simulink model "AN_Simulink_Model_v1_fil"  (R2019b)
settings: Solver=VariableStepAuto  StartTime=0.0  StopTime=testtime  RelTol=1e-3
InitFcn:
  | AN_InitFcn_Callback
StopFcn:
  | AN_StopFcn_Callback
values from neighbouring files (symbols this model uses):
  tdres = 1/Fs    (= 2.08333333333e-05)    [AN_Set_Model_Parameters.m]
libraries: hdlmdlgenlib x163, simulink x4, fillib x1, dspsrcs4 x1
(part 3 of 5)

== system AN_Simulink_Model_v1_fil/Auditory Nerve Model/C2 Wideband Filter/Sum7 ==
  In1 : Inport
  In2 : Inport  Port=2
  Sum7 : Sum  OutDataTypeStr=single  SampleTime=2.08333333333333e-05  SaturateOnIntegerOverflow=on  InputSameDT=on
  Out1 : Outport
  wires:
  Sum7/1 -> Out1/1
  In2/1 -> Sum7/2
  In1/1 -> Sum7/1

== system AN_Simulink_Model_v1_fil/Auditory Nerve Model/C2 Wideband Filter/Sum8 ==
  In1 : Inport
  In2 : Inport  Port=2
  Sum8 : Sum  OutDataTypeStr=single  SampleTime=2.08333333333333e-05  SaturateOnIntegerOverflow=on  InputSameDT=on
  Out1 : Outport
  wires:
  Sum8/1 -> Out1/1
  In2/1 -> Sum8/2
  In1/1 -> Sum8/1

== system AN_Simulink_Model_v1_fil/Auditory Nerve Model/C2 Wideband Filter/Sum9 ==
  In1 : Inport
  In2 : Inport  Port=2
  Sum9 : Sum  OutDataTypeStr=single  SampleTime=2.08333333333333e-05  SaturateOnIntegerOverflow=on  InputSameDT=on
  Out1 : Outport
  wires:
  Sum9/1 -> Out1/1
  In2/1 -> Sum9/2
  In1/1 -> Sum9/1

== system AN_Simulink_Model_v1_fil/Auditory Nerve Model/Middle Ear Filter/Gain1_unaryminus ==
  In1 : Inport
  Gain1_unaryminus : UnaryMinus  SampleTime=2.08333333333333e-05
  Out1 : Outport
  wires:
  Gain1_unaryminus/1 -> Out1/1
  In1/1 -> Gain1_unaryminus/1

== system AN_Simulink_Model_v1_fil/Auditory Nerve Model/Middle Ear Filter/Gain2_unaryminus ==
  In1 : Inport
  Gain2_unaryminus : UnaryMinus  SampleTime=2.08333333333333e-05
  Out1 : Outport
  wires:
  Gain2_unaryminus/1 -> Out1/1
  In1/1 -> Gain2_unaryminus/1

== system AN_Simulink_Model_v1_fil/Auditory Nerve Model/Middle Ear Filter/Gain3_unaryminus ==
  In1 : Inport
  Gain3_unaryminus : UnaryMinus  SampleTime=2.08333333333333e-05
  Out1 : Outport
  wires:
  Gain3_unaryminus/1 -> Out1/1
  In1/1 -> Gain3_unaryminus/1

== system AN_Simulink_Model_v1_fil/Auditory Nerve Model/Middle Ear Filter/Gain5_unaryminus ==
  In1 : Inport
  Gain5_unaryminus : UnaryMinus  SampleTime=2.08333333333333e-05
  Out1 : Outport
  wires:
  Gain5_unaryminus/1 -> Out1/1
  In1/1 -> Gain5_unaryminus/1

== system AN_Simulink_Model_v1_fil/Auditory Nerve Model/Middle Ear Filter/Gain7_unaryminus ==
  In1 : Inport
  Gain7_unaryminus : UnaryMinus  SampleTime=2.08333333333333e-05
  Out1 : Outport
  wires:
  Gain7_unaryminus/1 -> Out1/1
  In1/1 -> Gain7_unaryminus/1

== system AN_Simulink_Model_v1_fil/Auditory Nerve Model/Middle Ear Filter/Gain8_unaryminus ==
  In1 : Inport
  Gain8_unaryminus : UnaryMinus  SampleTime=2.08333333333333e-05
  Out1 : Outport
  wires:
  Gain8_unaryminus/1 -> Out1/1
  In1/1 -> Gain8_unaryminus/1

== system AN_Simulink_Model_v1_fil/Auditory Nerve Model/Middle Ear Filter/Product ==
  In1 : Inport
  In2 : Inport  Port=2
  Product : Product  Inputs=**  OutDataTypeStr=single  SampleTime=2.08333333333333e-05
  Out1 : Outport
  wires:
  Product/1 -> Out1/1
  In2/1 -> Product/2
  In1/1 -> Product/1

== system AN_Simulink_Model_v1_fil/Auditory Nerve Model/Middle Ear Filter/Product1 ==
  In1 : Inport
  In2 : Inport  Port=2
  Product1 : Product  Inputs=**  OutDataTypeStr=single  SampleTime=2.08333333333333e-05
  Out1 : Outport
  wires:
  Product1/1 -> Out1/1
  In2/1 -> Product1/2
  In1/1 -> Product1/1

== system AN_Simulink_Model_v1_fil/Auditory Nerve Model/Middle Ear Filter/Product10 ==
  In1 : Inport
  In2 : Inport  Port=2
  Product10 : Product  Inputs=**  OutDataTypeStr=single  SampleTime=2.08333333333333e-05
  Out1 : Outport
  wires:
  Product10/1 -> Out1/1
  In2/1 -> Product10/2
  In1/1 -> Product10/1

== system AN_Simulink_Model_v1_fil/Auditory Nerve Model/Middle Ear Filter/Product11 ==
  In1 : Inport
  In2 : Inport  Port=2
  Product11 : Product  Inputs=**  OutDataTypeStr=single  SampleTime=2.08333333333333e-05
  Out1 : Outport
  wires:
  Product11/1 -> Out1/1
  In2/1 -> Product11/2
  In1/1 -> Product11/1

== system AN_Simulink_Model_v1_fil/Auditory Nerve Model/Middle Ear Filter/Product12 ==
  In1 : Inport
  In2 : Inport  Port=2
  Product12 : Product  Inputs=**  OutDataTypeStr=single  SampleTime=2.08333333333333e-05
  Out1 : Outport
  wires:
  Product12/1 -> Out1/1
  In2/1 -> Product12/2
  In1/1 -> Product12/1

== system AN_Simulink_Model_v1_fil/Auditory Nerve Model/Middle Ear Filter/Product13 ==
  In1 : Inport
  In2 : Inport  Port=2
  Product13 : Product  Inputs=**  OutDataTypeStr=single  SampleTime=2.08333333333333e-05
  Out1 : Outport
  wires:
  Product13/1 -> Out1/1
  In2/1 -> Product13/2
  In1/1 -> Product13/1

== system AN_Simulink_Model_v1_fil/Auditory Nerve Model/Middle Ear Filter/Product14 ==
  In1 : Inport
  In2 : Inport  Port=2
  Product14 : Product  Inputs=**  OutDataTypeStr=single  SampleTime=2.08333333333333e-05
  Out1 : Outport
  wires:
  Product14/1 -> Out1/1
  In2/1 -> Product14/2
  In1/1 -> Product14/1

== system AN_Simulink_Model_v1_fil/Auditory Nerve Model/Middle Ear Filter/Product15_to_gain ==
  In1 : Inport
  Product15_to_gain : Gain  Gain=single(0.5)
  Out1 : Outport
  wires:
  Product15_to_gain/1 -> Out1/1
  In1/1 -> Product15_to_gain/1

== system AN_Simulink_Model_v1_fil/Auditory Nerve Model/Middle Ear Filter/Product2 ==
  In1 : Inport
  In2 : Inport  Port=2
  Product2 : Product  Inputs=**  OutDataTypeStr=single  SampleTime=2.08333333333333e-05
  Out1 : Outport
  wires:
  Product2/1 -> Out1/1
  In2/1 -> Product2/2
  In1/1 -> Product2/1

== system AN_Simulink_Model_v1_fil/Auditory Nerve Model/Middle Ear Filter/Product3 ==
  In1 : Inport
  In2 : Inport  Port=2
  Product3 : Product  Inputs=**  OutDataTypeStr=single  SampleTime=2.08333333333333e-05
  Out1 : Outport
  wires:
  Product3/1 -> Out1/1
  In2/1 -> Product3/2
  In1/1 -> Product3/1

== system AN_Simulink_Model_v1_fil/Auditory Nerve Model/Middle Ear Filter/Product4 ==
  In1 : Inport
  In2 : Inport  Port=2
  Product4 : Product  Inputs=**  OutDataTypeStr=single  SampleTime=2.08333333333333e-05
  Out1 : Outport
  wires:
  Product4/1 -> Out1/1
  In2/1 -> Product4/2
  In1/1 -> Product4/1

== system AN_Simulink_Model_v1_fil/Auditory Nerve Model/Middle Ear Filter/Product5 ==
  In1 : Inport
  In2 : Inport  Port=2
  Product5 : Product  Inputs=**  OutDataTypeStr=single  SampleTime=2.08333333333333e-05
  Out1 : Outport
  wires:
  Product5/1 -> Out1/1
  In2/1 -> Product5/2
  In1/1 -> Product5/1

== system AN_Simulink_Model_v1_fil/Auditory Nerve Model/Middle Ear Filter/Product6 ==
  In1 : Inport
  In2 : Inport  Port=2
  Product6 : Product  Inputs=**  OutDataTypeStr=single  SampleTime=2.08333333333333e-05
  Out1 : Outport
  wires:
  Product6/1 -> Out1/1
  In2/1 -> Product6/2
  In1/1 -> Product6/1

== system AN_Simulink_Model_v1_fil/Auditory Nerve Model/Middle Ear Filter/Product7 ==
  In1 : Inport
  In2 : Inport  Port=2
  Product7 : Product  Inputs=**  OutDataTypeStr=single  SampleTime=2.08333333333333e-05
  Out1 : Outport
  wires:
  Product7/1 -> Out1/1
  In2/1 -> Product7/2
  In1/1 -> Product7/1

== system AN_Simulink_Model_v1_fil/Auditory Nerve Model/Middle Ear Filter/Product8 ==
  In1 : Inport
  In2 : Inport  Port=2
  Product8 : Product  Inputs=**  OutDataTypeStr=single  SampleTime=2.08333333333333e-05
  Out1 : Outport
  wires:
  Product8/1 -> Out1/1
  In2/1 -> Product8/2
  In1/1 -> Product8/1

== system AN_Simulink_Model_v1_fil/Auditory Nerve Model/Middle Ear Filter/Product9 ==
  In1 : Inport
  In2 : Inport  Port=2
  Product9 : Product  Inputs=**  OutDataTypeStr=single  SampleTime=2.08333333333333e-05
  Out1 : Outport
  wires:
  Product9/1 -> Out1/1
  In2/1 -> Product9/2
  In1/1 -> Product9/1

== system AN_Simulink_Model_v1_fil/Auditory Nerve Model/Middle Ear Filter/Sum ==
  In1 : Inport
  In2 : Inport  Port=2
  Sum : Sum  OutDataTypeStr=single  SampleTime=2.08333333333333e-05  SaturateOnIntegerOverflow=on  InputSameDT=on
  Out1 : Outport
  wires:
  Sum/1 -> Out1/1
  In2/1 -> Sum/2
  In1/1 -> Sum/1

== system AN_Simulink_Model_v1_fil/Auditory Nerve Model/Middle Ear Filter/Sum1 ==
  In1 : Inport
  In2 : Inport  Port=2
  Sum1 : Sum  OutDataTypeStr=single  SampleTime=2.08333333333333e-05  SaturateOnIntegerOverflow=on  InputSameDT=on
  Out1 : Outport
  wires:
  Sum1/1 -> Out1/1
  In2/1 -> Sum1/2
  In1/1 -> Sum1/1

== system AN_Simulink_Model_v1_fil/Auditory Nerve Model/Middle Ear Filter/Sum10 ==
  In1 : Inport
  In2 : Inport  Port=2
  Sum10 : Sum  OutDataTypeStr=single  SampleTime=2.08333333333333e-05  SaturateOnIntegerOverflow=on  InputSameDT=on
  Out1 : Outport
  wires:
  Sum10/1 -> Out1/1
  In2/1 -> Sum10/2
  In1/1 -> Sum10/1

== system AN_Simulink_Model_v1_fil/Auditory Nerve Model/Middle Ear Filter/Sum11 ==
  In1 : Inport
  In2 : Inport  Port=2
  Sum11 : Sum  OutDataTypeStr=single  SampleTime=2.08333333333333e-05  SaturateOnIntegerOverflow=on  InputSameDT=on
  Out1 : Outport
  wires:
  Sum11/1 -> Out1/1
  In2/1 -> Sum11/2
  In1/1 -> Sum11/1

== system AN_Simulink_Model_v1_fil/Auditory Nerve Model/Middle Ear Filter/Sum2 ==
  In1 : Inport
  In2 : Inport  Port=2
  Sum2 : Sum  OutDataTypeStr=single  SampleTime=2.08333333333333e-05  SaturateOnIntegerOverflow=on  InputSameDT=on
  Out1 : Outport
  wires:
  Sum2/1 -> Out1/1
  In2/1 -> Sum2/2
  In1/1 -> Sum2/1

== system AN_Simulink_Model_v1_fil/Auditory Nerve Model/Middle Ear Filter/Sum3 ==
  In1 : Inport
  In2 : Inport  Port=2
  Sum3 : Sum  OutDataTypeStr=single  SampleTime=2.08333333333333e-05  SaturateOnIntegerOverflow=on  InputSameDT=on
  Out1 : Outport
  wires:
  Sum3/1 -> Out1/1
  In2/1 -> Sum3/2
  In1/1 -> Sum3/1

== system AN_Simulink_Model_v1_fil/Auditory Nerve Model/Middle Ear Filter/Sum4 ==
  In1 : Inport
  In2 : Inport  Port=2
  Sum4 : Sum  OutDataTypeStr=single  SampleTime=2.08333333333333e-05  SaturateOnIntegerOverflow=on  InputSameDT=on
  Out1 : Outport
  wires:
  Sum4/1 -> Out1/1
  In2/1 -> Sum4/2
  In1/1 -> Sum4/1

== system AN_Simulink_Model_v1_fil/Auditory Nerve Model/Middle Ear Filter/Sum5 ==
  In1 : Inport
  In2 : Inport  Port=2
  Sum5 : Sum  OutDataTypeStr=single  SampleTime=2.08333333333333e-05  SaturateOnIntegerOverflow=on  InputSameDT=on
  Out1 : Outport
  wires:
  Sum5/1 -> Out1/1
  In2/1 -> Sum5/2
  In1/1 -> Sum5/1

== system AN_Simulink_Model_v1_fil/Auditory Nerve Model/Middle Ear Filter/Sum6 ==
  In1 : Inport
  In2 : Inport  Port=2
  Sum6 : Sum  OutDataTypeStr=single  SampleTime=2.08333333333333e-05  SaturateOnIntegerOverflow=on  InputSameDT=on
  Out1 : Outport
  wires:
  Sum6/1 -> Out1/1
  In2/1 -> Sum6/2
  In1/1 -> Sum6/1

== system AN_Simulink_Model_v1_fil/Auditory Nerve Model/Middle Ear Filter/Sum7 ==
  In1 : Inport
  In2 : Inport  Port=2
  Sum7 : Sum  OutDataTypeStr=single  SampleTime=2.08333333333333e-05  SaturateOnIntegerOverflow=on  InputSameDT=on
  Out1 : Outport
  wires:
  Sum7/1 -> Out1/1
  In2/1 -> Sum7/2
  In1/1 -> Sum7/1

== system AN_Simulink_Model_v1_fil/Auditory Nerve Model/Middle Ear Filter/Sum8 ==
  In1 : Inport
  In2 : Inport  Port=2
  Sum8 : Sum  OutDataTypeStr=single  SampleTime=2.08333333333333e-05  SaturateOnIntegerOverflow=on  InputSameDT=on
  Out1 : Outport
  wires:
  Sum8/1 -> Out1/1
  In2/1 -> Sum8/2
  In1/1 -> Sum8/1

== system AN_Simulink_Model_v1_fil/Auditory Nerve Model/Middle Ear Filter/Sum9 ==
  In1 : Inport
  In2 : Inport  Port=2
  Sum9 : Sum  OutDataTypeStr=single  SampleTime=2.08333333333333e-05  SaturateOnIntegerOverflow=on  InputSameDT=on
  Out1 : Outport
  wires:
  Sum9/1 -> Out1/1
  In2/1 -> Sum9/2
  In1/1 -> Sum9/1

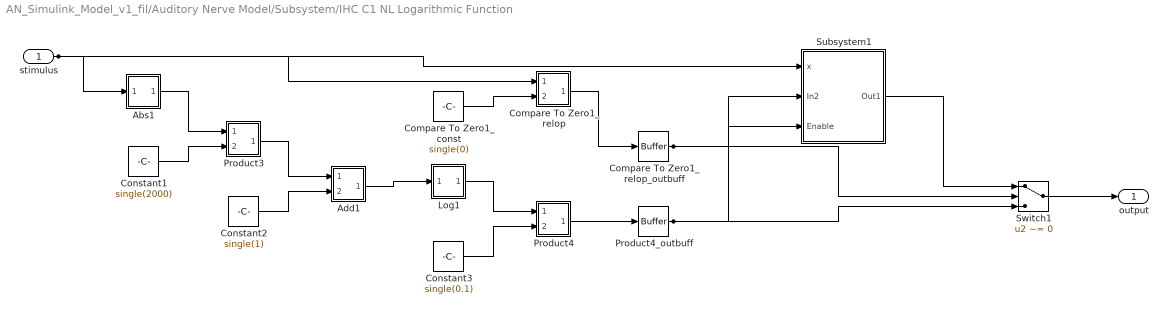
== system AN_Simulink_Model_v1_fil/Auditory Nerve Model/Subsystem/IHC C1 NL Logarithmic Function ==
  stimulus : Inport  OutDataTypeStr=single  PortDimensions=1  SampleTime=2.08333333333333e-05
  Abs1 : Subsystem
      mask Display: disp('NFP\nabs');
  Add1 : Subsystem
      mask Display: disp('NFP\nadd');
  Compare To Zero1_const : Constant  Value=single(0)  OutDataTypeStr=single  SampleTime=-1
  Compare To Zero1_relop : Subsystem
      mask Display: disp('NFP\nrelop');
  Compare To Zero1_relop_outbuff : hdlmdlgenlib/Buffer
      settings: SourceProductName=Simulink  SourceProductBaseCode=SL
  Constant1 : Constant  Value=single(2000)  OutDataTypeStr=single  SampleTime=-1
  Constant2 : Constant  Value=single(1)  OutDataTypeStr=single  SampleTime=-1
  Constant3 : Constant  Value=single(0.1)  OutDataTypeStr=single  SampleTime=-1
  Log1 : Subsystem
      mask Display: disp('NFP\nmath');
  Product3 : Subsystem
      mask Display: disp('NFP\nmul');
  Product4 : Subsystem
      mask Display: disp('NFP\nmul');
  Product4_outbuff : hdlmdlgenlib/Buffer
      settings: SourceProductName=Simulink  SourceProductBaseCode=SL
  Subsystem1 : Subsystem
  Switch1 : Switch  Criteria=u2 ~= 0  Threshold=double(0)  OutDataTypeStr=single  SampleTime=2.08333333333333e-05
  output : Outport  VectorParamsAs1DForOutWhenUnconnected=off
  wires:
  Product4/1(Out1) -> Product4_outbuff/1
  Product3/1(Out1) -> Add1/1(In1)
  Log1/1(Out1) -> Product4/1(In1)
  Compare To Zero1_relop/1(Out1) -> Compare To Zero1_relop_outbuff/1
  Add1/1(Out1) -> Log1/1(In1)
  Abs1/1(Out1) -> Product3/1(In1)
  Compare To Zero1_const/1 -> Compare To Zero1_relop/2(In2)
  Switch1/1 -> output/1
  Subsystem1/1(Out1) -> Switch1/1
  Product4_outbuff/1 -> Subsystem1/2(In2), Switch1/3
  Constant3/1 -> Product4/2(In2)
  Constant2/1 -> Add1/2(In2)
  Constant1/1 -> Product3/2(In2)
  Compare To Zero1_relop_outbuff/1 -> Subsystem1/3(Enable), Switch1/2
  stimulus/1 -> Subsystem1/1(x), Abs1/1(In1), Compare To Zero1_relop/1(In1)

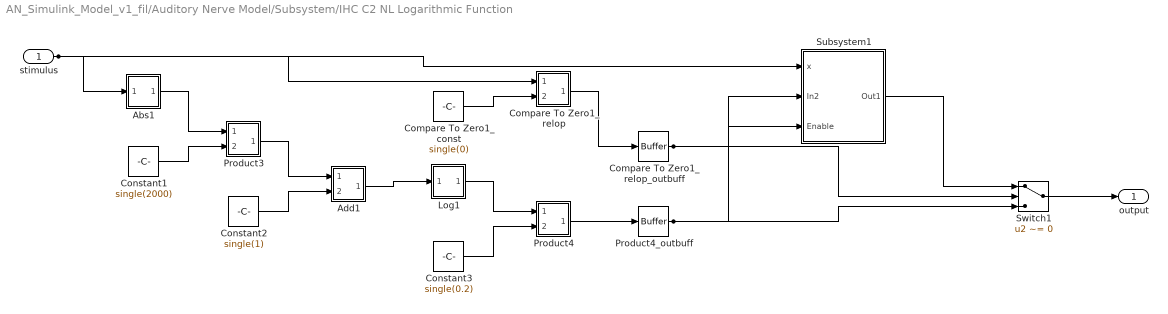
== system AN_Simulink_Model_v1_fil/Auditory Nerve Model/Subsystem/IHC C2 NL Logarithmic Function ==
  stimulus : Inport  OutDataTypeStr=single  PortDimensions=1  SampleTime=2.08333333333333e-05
  Abs1 : Subsystem
      mask Display: disp('NFP\nabs');
  Add1 : Subsystem
      mask Display: disp('NFP\nadd');
  Compare To Zero1_const : Constant  Value=single(0)  OutDataTypeStr=single  SampleTime=-1
  Compare To Zero1_relop : Subsystem
      mask Display: disp('NFP\nrelop');
  Compare To Zero1_relop_outbuff : hdlmdlgenlib/Buffer
      settings: SourceProductName=Simulink  SourceProductBaseCode=SL
  Constant1 : Constant  Value=single(2000)  OutDataTypeStr=single  SampleTime=-1
  Constant2 : Constant  Value=single(1)  OutDataTypeStr=single  SampleTime=-1
  Constant3 : Constant  Value=single(0.2)  OutDataTypeStr=single  SampleTime=-1
  Log1 : Subsystem
      mask Display: disp('NFP\nmath');
  Product3 : Subsystem
      mask Display: disp('NFP\nmul');
  Product4 : Subsystem
      mask Display: disp('NFP\nmul');
  Product4_outbuff : hdlmdlgenlib/Buffer
      settings: SourceProductName=Simulink  SourceProductBaseCode=SL
  Subsystem1 : Subsystem
  Switch1 : Switch  Criteria=u2 ~= 0  Threshold=double(0)  OutDataTypeStr=single  SampleTime=2.08333333333333e-05
  output : Outport  VectorParamsAs1DForOutWhenUnconnected=off
  wires:
  Product4/1(Out1) -> Product4_outbuff/1
  Product3/1(Out1) -> Add1/1(In1)
  Log1/1(Out1) -> Product4/1(In1)
  Compare To Zero1_relop/1(Out1) -> Compare To Zero1_relop_outbuff/1
  Add1/1(Out1) -> Log1/1(In1)
  Abs1/1(Out1) -> Product3/1(In1)
  Compare To Zero1_const/1 -> Compare To Zero1_relop/2(In2)
  Switch1/1 -> output/1
  Subsystem1/1(Out1) -> Switch1/1
  Product4_outbuff/1 -> Subsystem1/2(In2), Switch1/3
  Constant3/1 -> Product4/2(In2)
  Constant2/1 -> Add1/2(In2)
  Constant1/1 -> Product3/2(In2)
  Compare To Zero1_relop_outbuff/1 -> Subsystem1/3(Enable), Switch1/2
  stimulus/1 -> Subsystem1/1(x), Abs1/1(In1), Compare To Zero1_relop/1(In1)

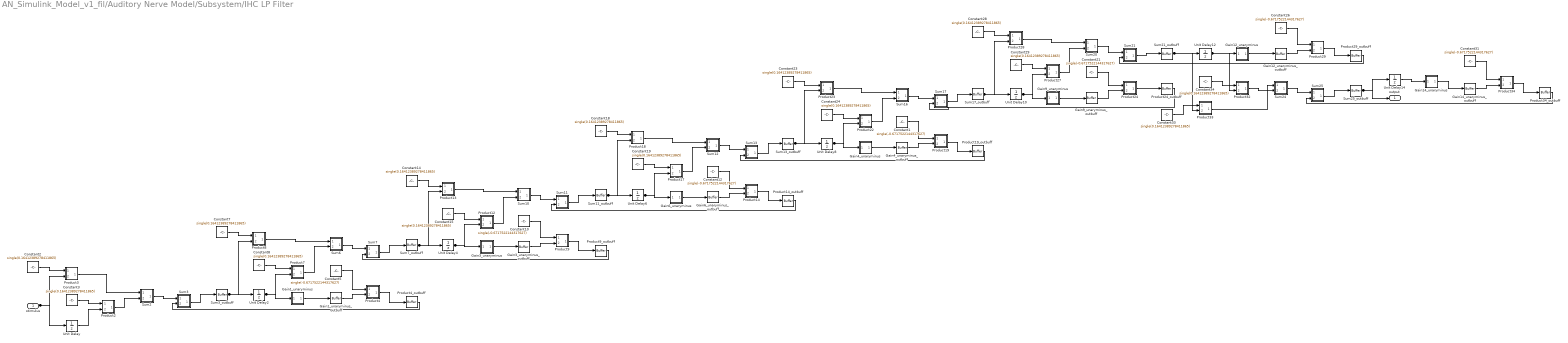
== system AN_Simulink_Model_v1_fil/Auditory Nerve Model/Subsystem/IHC LP Filter ==
  stimulus : Inport  OutDataTypeStr=single  PortDimensions=1  SampleTime=2.08333333333333e-05
  Constant{1,5,10,12,21,26,31} (7 alike) : Constant  Value=single(-0.6717522144317627)  OutDataTypeStr=single  SampleTime=-1
  Constant{2..3,7..8,14..15,18..19,23..24,28..29,33..34} (14 alike) : Constant  Value=single(0.16412389278411865)  OutDataTypeStr=single  SampleTime=-1
  Gain12_unaryminus : Subsystem
      mask Display: disp('NFP\numinus');
  Gain12_unaryminus_outbuff : hdlmdlgenlib/Buffer
      settings: SourceProductName=Simulink  SourceProductBaseCode=SL
  Gain14_unaryminus : Subsystem
      mask Display: disp('NFP\numinus');
  Gain14_unaryminus_outbuff : hdlmdlgenlib/Buffer
      settings: SourceProductName=Simulink  SourceProductBaseCode=SL
  Gain1_unaryminus : Subsystem
      mask Display: disp('NFP\numinus');
  Gain1_unaryminus_outbuff : hdlmdlgenlib/Buffer
      settings: SourceProductName=Simulink  SourceProductBaseCode=SL
  Gain3_unaryminus : Subsystem
      mask Display: disp('NFP\numinus');
  Gain3_unaryminus_outbuff : hdlmdlgenlib/Buffer
      settings: SourceProductName=Simulink  SourceProductBaseCode=SL
  Gain4_unaryminus : Subsystem
      mask Display: disp('NFP\numinus');
  Gain4_unaryminus_outbuff : hdlmdlgenlib/Buffer
      settings: SourceProductName=Simulink  SourceProductBaseCode=SL
  Gain6_unaryminus : Subsystem
      mask Display: disp('NFP\numinus');
  Gain6_unaryminus_outbuff : hdlmdlgenlib/Buffer
      settings: SourceProductName=Simulink  SourceProductBaseCode=SL
  Gain9_unaryminus : Subsystem
      mask Display: disp('NFP\numinus');
  Gain9_unaryminus_outbuff : hdlmdlgenlib/Buffer
      settings: SourceProductName=Simulink  SourceProductBaseCode=SL
  Product12 : Subsystem
      mask Display: disp('NFP\nmul');
  Product13 : Subsystem
      mask Display: disp('NFP\nmul');
  Product14 : Subsystem
      mask Display: disp('NFP\nmul');
  Product14_outbuff : hdlmdlgenlib/Buffer
      settings: SourceProductName=Simulink  SourceProductBaseCode=SL
  Product17 : Subsystem
      mask Display: disp('NFP\nmul');
  Product18 : Subsystem
      mask Display: disp('NFP\nmul');
  Product19 : Subsystem
      mask Display: disp('NFP\nmul');
  Product19_outbuff : hdlmdlgenlib/Buffer
      settings: SourceProductName=Simulink  SourceProductBaseCode=SL
  Product2 : Subsystem
      mask Display: disp('NFP\nmul');
  Product22 : Subsystem
      mask Display: disp('NFP\nmul');
  Product23 : Subsystem
      mask Display: disp('NFP\nmul');
  Product24 : Subsystem
      mask Display: disp('NFP\nmul');
  Product24_outbuff : hdlmdlgenlib/Buffer
      settings: SourceProductName=Simulink  SourceProductBaseCode=SL
  Product27 : Subsystem
      mask Display: disp('NFP\nmul');
  Product28 : Subsystem
      mask Display: disp('NFP\nmul');
  Product29 : Subsystem
      mask Display: disp('NFP\nmul');
  Product29_outbuff : hdlmdlgenlib/Buffer
      settings: SourceProductName=Simulink  SourceProductBaseCode=SL
  Product3 : Subsystem
      mask Display: disp('NFP\nmul');
  Product32 : Subsystem
      mask Display: disp('NFP\nmul');
  Product33 : Subsystem
      mask Display: disp('NFP\nmul');
  Product34 : Subsystem
      mask Display: disp('NFP\nmul');
  Product34_outbuff : hdlmdlgenlib/Buffer
      settings: SourceProductName=Simulink  SourceProductBaseCode=SL
  Product4 : Subsystem
      mask Display: disp('NFP\nmul');
  Product4_outbuff : hdlmdlgenlib/Buffer
      settings: SourceProductName=Simulink  SourceProductBaseCode=SL
  Product7 : Subsystem
      mask Display: disp('NFP\nmul');
  Product8 : Subsystem
      mask Display: disp('NFP\nmul');
  Product9 : Subsystem
      mask Display: disp('NFP\nmul');
  Product9_outbuff : hdlmdlgenlib/Buffer
      settings: SourceProductName=Simulink  SourceProductBaseCode=SL
  Sum10 : Subsystem
      mask Display: disp('NFP\nadd');
  Sum11 : Subsystem
      mask Display: disp('NFP\nadd');
  Sum11_outbuff : hdlmdlgenlib/Buffer
      settings: SourceProductName=Simulink  SourceProductBaseCode=SL
  Sum12 : Subsystem
      mask Display: disp('NFP\nadd');
  Sum13 : Subsystem
      mask Display: disp('NFP\nadd');
  Sum13_outbuff : hdlmdlgenlib/Buffer
      settings: SourceProductName=Simulink  SourceProductBaseCode=SL
  Sum16 : Subsystem
      mask Display: disp('NFP\nadd');
  Sum17 : Subsystem
      mask Display: disp('NFP\nadd');
  Sum17_outbuff : hdlmdlgenlib/Buffer
      settings: SourceProductName=Simulink  SourceProductBaseCode=SL
  Sum2 : Subsystem
      mask Display: disp('NFP\nadd');
  Sum20 : Subsystem
      mask Display: disp('NFP\nadd');
  Sum21 : Subsystem
      mask Display: disp('NFP\nadd');
  Sum21_outbuff : hdlmdlgenlib/Buffer
      settings: SourceProductName=Simulink  SourceProductBaseCode=SL
  Sum24 : Subsystem
      mask Display: disp('NFP\nadd');
  Sum25 : Subsystem
      mask Display: disp('NFP\nadd');
  Sum25_outbuff : hdlmdlgenlib/Buffer
      settings: SourceProductName=Simulink  SourceProductBaseCode=SL
  Sum3 : Subsystem
      mask Display: disp('NFP\nadd');
  Sum3_outbuff : hdlmdlgenlib/Buffer
      settings: SourceProductName=Simulink  SourceProductBaseCode=SL
  Sum6 : Subsystem
      mask Display: disp('NFP\nadd');
  Sum7 : Subsystem
      mask Display: disp('NFP\nadd');
  Sum7_outbuff : hdlmdlgenlib/Buffer
      settings: SourceProductName=Simulink  SourceProductBaseCode=SL
  Unit Delay{,2,4,6,8,10,12,14} (8 alike) : UnitDelay  InitialCondition=single(0)  SampleTime=2.08333333333333e-05
  output : Outport  VectorParamsAs1DForOutWhenUnconnected=off
  wires:
  Sum7/1(Out1) -> Sum7_outbuff/1
  Sum6/1(Out1) -> Sum7/1(In1)
  Sum3/1(Out1) -> Sum3_outbuff/1
  Sum25/1(Out1) -> Sum25_outbuff/1
  Sum24/1(Out1) -> Sum25/1(In1)
  Sum21/1(Out1) -> Sum21_outbuff/1
  Sum20/1(Out1) -> Sum21/1(In1)
  Sum2/1(Out1) -> Sum3/1(In1)
  Sum17/1(Out1) -> Sum17_outbuff/1
  Sum16/1(Out1) -> Sum17/1(In1)
  Sum13/1(Out1) -> Sum13_outbuff/1
  Sum12/1(Out1) -> Sum13/1(In1)
  Sum11/1(Out1) -> Sum11_outbuff/1
  Sum10/1(Out1) -> Sum11/1(In1)
  Product9/1(Out1) -> Product9_outbuff/1
  Product8/1(Out1) -> Sum6/1(In1)
  Product7/1(Out1) -> Sum6/2(In2)
  Product4/1(Out1) -> Product4_outbuff/1
  Product34/1(Out1) -> Product34_outbuff/1
  Product33/1(Out1) -> Sum24/1(In1)
  Product32/1(Out1) -> Sum24/2(In2)
  Product3/1(Out1) -> Sum2/1(In1)
  Product29/1(Out1) -> Product29_outbuff/1
  Product28/1(Out1) -> Sum20/1(In1)
  Product27/1(Out1) -> Sum20/2(In2)
  Product24/1(Out1) -> Product24_outbuff/1
  Product23/1(Out1) -> Sum16/1(In1)
  Product22/1(Out1) -> Sum16/2(In2)
  Product2/1(Out1) -> Sum2/2(In2)
  Product19/1(Out1) -> Product19_outbuff/1
  Product18/1(Out1) -> Sum12/1(In1)
  Product17/1(Out1) -> Sum12/2(In2)
  Product14/1(Out1) -> Product14_outbuff/1
  Product13/1(Out1) -> Sum10/1(In1)
  Product12/1(Out1) -> Sum10/2(In2)
  Gain9_unaryminus/1(Out1) -> Gain9_unaryminus_outbuff/1
  Gain6_unaryminus/1(Out1) -> Gain6_unaryminus_outbuff/1
  Gain4_unaryminus/1(Out1) -> Gain4_unaryminus_outbuff/1
  Gain3_unaryminus/1(Out1) -> Gain3_unaryminus_outbuff/1
  Gain14_unaryminus/1(Out1) -> Gain14_unaryminus_outbuff/1
  Gain12_unaryminus/1(Out1) -> Gain12_unaryminus_outbuff/1
  Gain1_unaryminus/1(Out1) -> Gain1_unaryminus_outbuff/1
  Unit Delay8/1 -> Gain4_unaryminus/1(In1), Product22/2(In2)
  Unit Delay6/1 -> Gain6_unaryminus/1(In1), Product17/2(In2)
  Unit Delay4/1 -> Gain3_unaryminus/1(In1), Product12/2(In2)
  Unit Delay2/1 -> Gain1_unaryminus/1(In1), Product7/2(In2)
  Unit Delay14/1 -> Gain14_unaryminus/1(In1)
  Unit Delay12/1 -> Gain12_unaryminus/1(In1), Product32/2(In2)
  Unit Delay10/1 -> Gain9_unaryminus/1(In1), Product27/2(In2)
  Unit Delay/1 -> Product2/2(In2)
  Sum7_outbuff/1 -> Unit Delay4/1, Product13/2(In2)
  Sum3_outbuff/1 -> Unit Delay2/1, Product8/2(In2)
  Sum25_outbuff/1 -> output/1, Unit Delay14/1
  Sum21_outbuff/1 -> Unit Delay12/1, Product33/2(In2)
  Sum17_outbuff/1 -> Unit Delay10/1, Product28/2(In2)
  Sum13_outbuff/1 -> Unit Delay8/1, Product23/2(In2)
  Sum11_outbuff/1 -> Unit Delay6/1, Product18/2(In2)
  Product9_outbuff/1 -> Sum7/2(In2)
  Product4_outbuff/1 -> Sum3/2(In2)
  Product34_outbuff/1 -> Sum25/2(In2)
  Product29_outbuff/1 -> Sum21/2(In2)
  Product24_outbuff/1 -> Sum17/2(In2)
  Product19_outbuff/1 -> Sum13/2(In2)
  Product14_outbuff/1 -> Sum11/2(In2)
  Gain9_unaryminus_outbuff/1 -> Product24/2(In2)
  Gain6_unaryminus_outbuff/1 -> Product14/2(In2)
  Gain4_unaryminus_outbuff/1 -> Product19/2(In2)
  Gain3_unaryminus_outbuff/1 -> Product9/2(In2)
  Gain14_unaryminus_outbuff/1 -> Product34/2(In2)
  Gain12_unaryminus_outbuff/1 -> Product29/2(In2)
  Gain1_unaryminus_outbuff/1 -> Product4/2(In2)
  Constant8/1 -> Product7/1(In1)
  Constant7/1 -> Product8/1(In1)
  Constant5/1 -> Product4/1(In1)
  Constant34/1 -> Product32/1(In1)
  Constant33/1 -> Product33/1(In1)
  Constant31/1 -> Product34/1(In1)
  Constant3/1 -> Product2/1(In1)
  Constant29/1 -> Product27/1(In1)
  Constant28/1 -> Product28/1(In1)
  Constant26/1 -> Product29/1(In1)
  Constant24/1 -> Product22/1(In1)
  Constant23/1 -> Product23/1(In1)
  Constant21/1 -> Product24/1(In1)
  Constant2/1 -> Product3/1(In1)
  Constant19/1 -> Product17/1(In1)
  Constant18/1 -> Product18/1(In1)
  Constant15/1 -> Product12/1(In1)
  Constant14/1 -> Product13/1(In1)
  Constant12/1 -> Product14/1(In1)
  Constant10/1 -> Product9/1(In1)
  Constant1/1 -> Product19/1(In1)
  stimulus/1 -> Unit Delay/1, Product3/2(In2)

== system AN_Simulink_Model_v1_fil/Auditory Nerve Model/Subsystem/Sum1 ==
  In1 : Inport
  In2 : Inport  Port=2
  Sum1 : Sum  OutDataTypeStr=single  SampleTime=2.08333333333333e-05  SaturateOnIntegerOverflow=on  InputSameDT=on
  Out1 : Outport
  wires:
  Sum1/1 -> Out1/1
  In2/1 -> Sum1/2
  In1/1 -> Sum1/1

== system AN_Simulink_Model_v1_fil/Compare/Assert_ihcout/RelErrCheck ==
  In1 : Inport
  In2 : Inport  Port=2
  "RelativeErrorCheck " : MATLAB Function  TreatAsAtomicUnit=on
  Out1 : Outport  VectorParamsAs1DForOutWhenUnconnected=off
  wires:
  In2/1 -> "RelativeErrorCheck "/2(R)
  In1/1 -> "RelativeErrorCheck "/1(P)
  "RelativeErrorCheck "/1(y) -> Out1/1

== system AN_Simulink_Model_v1_fil/Auditory Nerve Model/C1 Chirp Filter/C1 FIlter/Gain10_unaryminus ==
  In1 : Inport
  Gain10_unaryminus : UnaryMinus  SampleTime=2.08333333333333e-05
  Out1 : Outport
  wires:
  Gain10_unaryminus/1 -> Out1/1
  In1/1 -> Gain10_unaryminus/1

== system AN_Simulink_Model_v1_fil/Auditory Nerve Model/C1 Chirp Filter/C1 FIlter/Gain11_unaryminus ==
  In1 : Inport
  Gain11_unaryminus : UnaryMinus  SampleTime=2.08333333333333e-05
  Out1 : Outport
  wires:
  Gain11_unaryminus/1 -> Out1/1
  In1/1 -> Gain11_unaryminus/1

== system AN_Simulink_Model_v1_fil/Auditory Nerve Model/C1 Chirp Filter/C1 FIlter/Gain1_unaryminus ==
  In1 : Inport
  Gain1_unaryminus : UnaryMinus  SampleTime=2.08333333333333e-05
  Out1 : Outport
  wires:
  Gain1_unaryminus/1 -> Out1/1
  In1/1 -> Gain1_unaryminus/1

== system AN_Simulink_Model_v1_fil/Auditory Nerve Model/C1 Chirp Filter/C1 FIlter/Gain2_unaryminus ==
  In1 : Inport
  Gain2_unaryminus : UnaryMinus  SampleTime=2.08333333333333e-05
  Out1 : Outport
  wires:
  Gain2_unaryminus/1 -> Out1/1
  In1/1 -> Gain2_unaryminus/1

== system AN_Simulink_Model_v1_fil/Auditory Nerve Model/C1 Chirp Filter/C1 FIlter/Gain3_unaryminus ==
  In1 : Inport
  Gain3_unaryminus : UnaryMinus  SampleTime=2.08333333333333e-05
  Out1 : Outport
  wires:
  Gain3_unaryminus/1 -> Out1/1
  In1/1 -> Gain3_unaryminus/1

== system AN_Simulink_Model_v1_fil/Auditory Nerve Model/C1 Chirp Filter/C1 FIlter/Gain4_unaryminus ==
  In1 : Inport
  Gain4_unaryminus : UnaryMinus  SampleTime=2.08333333333333e-05
  Out1 : Outport
  wires:
  Gain4_unaryminus/1 -> Out1/1
  In1/1 -> Gain4_unaryminus/1

== system AN_Simulink_Model_v1_fil/Auditory Nerve Model/C1 Chirp Filter/C1 FIlter/Gain5_unaryminus ==
  In1 : Inport
  Gain5_unaryminus : UnaryMinus  SampleTime=2.08333333333333e-05
  Out1 : Outport
  wires:
  Gain5_unaryminus/1 -> Out1/1
  In1/1 -> Gain5_unaryminus/1

== system AN_Simulink_Model_v1_fil/Auditory Nerve Model/C1 Chirp Filter/C1 FIlter/Gain7_unaryminus ==
  In1 : Inport
  Gain7_unaryminus : UnaryMinus  SampleTime=2.08333333333333e-05
  Out1 : Outport
  wires:
  Gain7_unaryminus/1 -> Out1/1
  In1/1 -> Gain7_unaryminus/1

== system AN_Simulink_Model_v1_fil/Auditory Nerve Model/C1 Chirp Filter/C1 FIlter/Gain8_unaryminus ==
  In1 : Inport
  Gain8_unaryminus : UnaryMinus  SampleTime=2.08333333333333e-05
  Out1 : Outport
  wires:
  Gain8_unaryminus/1 -> Out1/1
  In1/1 -> Gain8_unaryminus/1

== system AN_Simulink_Model_v1_fil/Auditory Nerve Model/C1 Chirp Filter/C1 FIlter/Gain9_unaryminus ==
  In1 : Inport
  Gain9_unaryminus : UnaryMinus  SampleTime=2.08333333333333e-05
  Out1 : Outport
  wires:
  Gain9_unaryminus/1 -> Out1/1
  In1/1 -> Gain9_unaryminus/1

== system AN_Simulink_Model_v1_fil/Auditory Nerve Model/C1 Chirp Filter/C1 FIlter/Product ==
  In1 : Inport
  In2 : Inport  Port=2
  Product : Product  Inputs=**  OutDataTypeStr=single  SampleTime=2.08333333333333e-05
  Out1 : Outport
  wires:
  Product/1 -> Out1/1
  In2/1 -> Product/2
  In1/1 -> Product/1

== system AN_Simulink_Model_v1_fil/Auditory Nerve Model/C1 Chirp Filter/C1 FIlter/Product1 ==
  In1 : Inport
  In2 : Inport  Port=2
  Product1 : Product  Inputs=**  OutDataTypeStr=single  SampleTime=2.08333333333333e-05
  Out1 : Outport
  wires:
  Product1/1 -> Out1/1
  In2/1 -> Product1/2
  In1/1 -> Product1/1

== system AN_Simulink_Model_v1_fil/Auditory Nerve Model/C1 Chirp Filter/C1 FIlter/Product10 ==
  In1 : Inport
  In2 : Inport  Port=2
  Product10 : Product  Inputs=**  OutDataTypeStr=single  SampleTime=2.08333333333333e-05
  Out1 : Outport
  wires:
  Product10/1 -> Out1/1
  In2/1 -> Product10/2
  In1/1 -> Product10/1

== system AN_Simulink_Model_v1_fil/Auditory Nerve Model/C1 Chirp Filter/C1 FIlter/Product11 ==
  In1 : Inport
  In2 : Inport  Port=2
  Product11 : Product  Inputs=**  OutDataTypeStr=single  SampleTime=2.08333333333333e-05
  Out1 : Outport
  wires:
  Product11/1 -> Out1/1
  In2/1 -> Product11/2
  In1/1 -> Product11/1

== system AN_Simulink_Model_v1_fil/Auditory Nerve Model/C1 Chirp Filter/C1 FIlter/Product12 ==
  In1 : Inport
  In2 : Inport  Port=2
  Product12 : Product  Inputs=**  OutDataTypeStr=single  SampleTime=2.08333333333333e-05
  Out1 : Outport
  wires:
  Product12/1 -> Out1/1
  In2/1 -> Product12/2
  In1/1 -> Product12/1

== system AN_Simulink_Model_v1_fil/Auditory Nerve Model/C1 Chirp Filter/C1 FIlter/Product13 ==
  In1 : Inport
  In2 : Inport  Port=2
  Product13 : Product  Inputs=**  OutDataTypeStr=single  SampleTime=2.08333333333333e-05
  Out1 : Outport
  wires:
  Product13/1 -> Out1/1
  In2/1 -> Product13/2
  In1/1 -> Product13/1

== system AN_Simulink_Model_v1_fil/Auditory Nerve Model/C1 Chirp Filter/C1 FIlter/Product14 ==
  In1 : Inport
  In2 : Inport  Port=2
  Product14 : Product  Inputs=**  OutDataTypeStr=single  SampleTime=2.08333333333333e-05
  Out1 : Outport
  wires:
  Product14/1 -> Out1/1
  In2/1 -> Product14/2
  In1/1 -> Product14/1

== system AN_Simulink_Model_v1_fil/Auditory Nerve Model/C1 Chirp Filter/C1 FIlter/Product15 ==
  In1 : Inport
  In2 : Inport  Port=2
  Product15 : Product  Inputs=**  OutDataTypeStr=single  SampleTime=2.08333333333333e-05
  Out1 : Outport
  wires:
  Product15/1 -> Out1/1
  In2/1 -> Product15/2
  In1/1 -> Product15/1

== system AN_Simulink_Model_v1_fil/Auditory Nerve Model/C1 Chirp Filter/C1 FIlter/Product16 ==
  In1 : Inport
  In2 : Inport  Port=2
  Product16 : Product  Inputs=**  OutDataTypeStr=single  SampleTime=2.08333333333333e-05
  Out1 : Outport
  wires:
  Product16/1 -> Out1/1
  In2/1 -> Product16/2
  In1/1 -> Product16/1

== system AN_Simulink_Model_v1_fil/Auditory Nerve Model/C1 Chirp Filter/C1 FIlter/Product17 ==
  In1 : Inport
  In2 : Inport  Port=2
  Product17 : Product  Inputs=**  OutDataTypeStr=single  SampleTime=2.08333333333333e-05
  Out1 : Outport
  wires:
  Product17/1 -> Out1/1
  In2/1 -> Product17/2
  In1/1 -> Product17/1

== system AN_Simulink_Model_v1_fil/Auditory Nerve Model/C1 Chirp Filter/C1 FIlter/Product18 ==
  In1 : Inport
  In2 : Inport  Port=2
  Product18 : Product  Inputs=**  OutDataTypeStr=single  SampleTime=2.08333333333333e-05
  Out1 : Outport
  wires:
  Product18/1 -> Out1/1
  In2/1 -> Product18/2
  In1/1 -> Product18/1

== system AN_Simulink_Model_v1_fil/Auditory Nerve Model/C1 Chirp Filter/C1 FIlter/Product19 ==
  In1 : Inport
  In2 : Inport  Port=2
  Product19 : Product  Inputs=**  OutDataTypeStr=single  SampleTime=2.08333333333333e-05
  Out1 : Outport
  wires:
  Product19/1 -> Out1/1
  In2/1 -> Product19/2
  In1/1 -> Product19/1

== system AN_Simulink_Model_v1_fil/Auditory Nerve Model/C1 Chirp Filter/C1 FIlter/Product2 ==
  In1 : Inport
  In2 : Inport  Port=2
  Product2 : Product  Inputs=**  OutDataTypeStr=single  SampleTime=2.08333333333333e-05
  Out1 : Outport
  wires:
  Product2/1 -> Out1/1
  In2/1 -> Product2/2
  In1/1 -> Product2/1

== system AN_Simulink_Model_v1_fil/Auditory Nerve Model/C1 Chirp Filter/C1 FIlter/Product20 ==
  In1 : Inport
  In2 : Inport  Port=2
  Product20 : Product  Inputs=**  OutDataTypeStr=single  SampleTime=2.08333333333333e-05
  Out1 : Outport
  wires:
  Product20/1 -> Out1/1
  In2/1 -> Product20/2
  In1/1 -> Product20/1

== system AN_Simulink_Model_v1_fil/Auditory Nerve Model/C1 Chirp Filter/C1 FIlter/Product21 ==
  In1 : Inport
  In2 : Inport  Port=2
  Product21 : Product  Inputs=**  OutDataTypeStr=single  SampleTime=2.08333333333333e-05
  Out1 : Outport
  wires:
  Product21/1 -> Out1/1
  In2/1 -> Product21/2
  In1/1 -> Product21/1

== system AN_Simulink_Model_v1_fil/Auditory Nerve Model/C1 Chirp Filter/C1 FIlter/Product22 ==
  In1 : Inport
  In2 : Inport  Port=2
  Product22 : Product  Inputs=**  OutDataTypeStr=single  SampleTime=2.08333333333333e-05
  Out1 : Outport
  wires:
  Product22/1 -> Out1/1
  In2/1 -> Product22/2
  In1/1 -> Product22/1

== system AN_Simulink_Model_v1_fil/Auditory Nerve Model/C1 Chirp Filter/C1 FIlter/Product23 ==
  In1 : Inport
  In2 : Inport  Port=2
  Product23 : Product  Inputs=**  OutDataTypeStr=single  SampleTime=2.08333333333333e-05
  Out1 : Outport
  wires:
  Product23/1 -> Out1/1
  In2/1 -> Product23/2
  In1/1 -> Product23/1

== system AN_Simulink_Model_v1_fil/Auditory Nerve Model/C1 Chirp Filter/C1 FIlter/Product24 ==
  In1 : Inport
  In2 : Inport  Port=2
  Product24 : Product  Inputs=**  OutDataTypeStr=single  SampleTime=2.08333333333333e-05
  Out1 : Outport
  wires:
  Product24/1 -> Out1/1
  In2/1 -> Product24/2
  In1/1 -> Product24/1

== system AN_Simulink_Model_v1_fil/Auditory Nerve Model/C1 Chirp Filter/C1 FIlter/Product25_to_gain ==
  In1 : Inport
  Product25_to_gain : Gain  Gain=single(0.25)
  Out1 : Outport
  wires:
  Product25_to_gain/1 -> Out1/1
  In1/1 -> Product25_to_gain/1

== system AN_Simulink_Model_v1_fil/Auditory Nerve Model/C1 Chirp Filter/C1 FIlter/Product26 ==
  In1 : Inport
  In2 : Inport  Port=2
  Product26 : Product  Inputs=**  OutDataTypeStr=single  SampleTime=2.08333333333333e-05
  Out1 : Outport
  wires:
  Product26/1 -> Out1/1
  In2/1 -> Product26/2
  In1/1 -> Product26/1

== system AN_Simulink_Model_v1_fil/Auditory Nerve Model/C1 Chirp Filter/C1 FIlter/Product3 ==
  In1 : Inport
  In2 : Inport  Port=2
  Product3 : Product  Inputs=**  OutDataTypeStr=single  SampleTime=2.08333333333333e-05
  Out1 : Outport
  wires:
  Product3/1 -> Out1/1
  In2/1 -> Product3/2
  In1/1 -> Product3/1

== system AN_Simulink_Model_v1_fil/Auditory Nerve Model/C1 Chirp Filter/C1 FIlter/Product4 ==
  In1 : Inport
  In2 : Inport  Port=2
  Product4 : Product  Inputs=**  OutDataTypeStr=single  SampleTime=2.08333333333333e-05
  Out1 : Outport
  wires:
  Product4/1 -> Out1/1
  In2/1 -> Product4/2
  In1/1 -> Product4/1

== system AN_Simulink_Model_v1_fil/Auditory Nerve Model/C1 Chirp Filter/C1 FIlter/Product5 ==
  In1 : Inport
  In2 : Inport  Port=2
  Product5 : Product  Inputs=**  OutDataTypeStr=single  SampleTime=2.08333333333333e-05
  Out1 : Outport
  wires:
  Product5/1 -> Out1/1
  In2/1 -> Product5/2
  In1/1 -> Product5/1

== system AN_Simulink_Model_v1_fil/Auditory Nerve Model/C1 Chirp Filter/C1 FIlter/Product6 ==
  In1 : Inport
  In2 : Inport  Port=2
  Product6 : Product  Inputs=**  OutDataTypeStr=single  SampleTime=2.08333333333333e-05
  Out1 : Outport
  wires:
  Product6/1 -> Out1/1
  In2/1 -> Product6/2
  In1/1 -> Product6/1

== system AN_Simulink_Model_v1_fil/Auditory Nerve Model/C1 Chirp Filter/C1 FIlter/Product7 ==
  In1 : Inport
  In2 : Inport  Port=2
  Product7 : Product  Inputs=**  OutDataTypeStr=single  SampleTime=2.08333333333333e-05
  Out1 : Outport
  wires:
  Product7/1 -> Out1/1
  In2/1 -> Product7/2
  In1/1 -> Product7/1

== system AN_Simulink_Model_v1_fil/Auditory Nerve Model/C1 Chirp Filter/C1 FIlter/Product8 ==
  In1 : Inport
  In2 : Inport  Port=2
  Product8 : Product  Inputs=**  OutDataTypeStr=single  SampleTime=2.08333333333333e-05
  Out1 : Outport
  wires:
  Product8/1 -> Out1/1
  In2/1 -> Product8/2
  In1/1 -> Product8/1

== system AN_Simulink_Model_v1_fil/Auditory Nerve Model/C1 Chirp Filter/C1 FIlter/Product9 ==
  In1 : Inport
  In2 : Inport  Port=2
  Product9 : Product  Inputs=**  OutDataTypeStr=single  SampleTime=2.08333333333333e-05
  Out1 : Outport
  wires:
  Product9/1 -> Out1/1
  In2/1 -> Product9/2
  In1/1 -> Product9/1

== system AN_Simulink_Model_v1_fil/Auditory Nerve Model/C1 Chirp Filter/C1 FIlter/Sum ==
  In1 : Inport
  In2 : Inport  Port=2
  Sum : Sum  OutDataTypeStr=single  SampleTime=2.08333333333333e-05  SaturateOnIntegerOverflow=on  InputSameDT=on
  Out1 : Outport
  wires:
  Sum/1 -> Out1/1
  In2/1 -> Sum/2
  In1/1 -> Sum/1

== system AN_Simulink_Model_v1_fil/Auditory Nerve Model/C1 Chirp Filter/C1 FIlter/Sum1 ==
  In1 : Inport
  In2 : Inport  Port=2
  Sum1 : Sum  OutDataTypeStr=single  SampleTime=2.08333333333333e-05  SaturateOnIntegerOverflow=on  InputSameDT=on
  Out1 : Outport
  wires:
  Sum1/1 -> Out1/1
  In2/1 -> Sum1/2
  In1/1 -> Sum1/1

== system AN_Simulink_Model_v1_fil/Auditory Nerve Model/C1 Chirp Filter/C1 FIlter/Sum10 ==
  In1 : Inport
  In2 : Inport  Port=2
  Sum10 : Sum  OutDataTypeStr=single  SampleTime=2.08333333333333e-05  SaturateOnIntegerOverflow=on  InputSameDT=on
  Out1 : Outport
  wires:
  Sum10/1 -> Out1/1
  In2/1 -> Sum10/2
  In1/1 -> Sum10/1

== system AN_Simulink_Model_v1_fil/Auditory Nerve Model/C1 Chirp Filter/C1 FIlter/Sum11 ==
  In1 : Inport
  In2 : Inport  Port=2
  Sum11 : Sum  OutDataTypeStr=single  SampleTime=2.08333333333333e-05  SaturateOnIntegerOverflow=on  InputSameDT=on
  Out1 : Outport
  wires:
  Sum11/1 -> Out1/1
  In2/1 -> Sum11/2
  In1/1 -> Sum11/1

== system AN_Simulink_Model_v1_fil/Auditory Nerve Model/C1 Chirp Filter/C1 FIlter/Sum12 ==
  In1 : Inport
  In2 : Inport  Port=2
  Sum12 : Sum  OutDataTypeStr=single  SampleTime=2.08333333333333e-05  SaturateOnIntegerOverflow=on  InputSameDT=on
  Out1 : Outport
  wires:
  Sum12/1 -> Out1/1
  In2/1 -> Sum12/2
  In1/1 -> Sum12/1

== system AN_Simulink_Model_v1_fil/Auditory Nerve Model/C1 Chirp Filter/C1 FIlter/Sum13 ==
  In1 : Inport
  In2 : Inport  Port=2
  Sum13 : Sum  OutDataTypeStr=single  SampleTime=2.08333333333333e-05  SaturateOnIntegerOverflow=on  InputSameDT=on
  Out1 : Outport
  wires:
  Sum13/1 -> Out1/1
  In2/1 -> Sum13/2
  In1/1 -> Sum13/1

== system AN_Simulink_Model_v1_fil/Auditory Nerve Model/C1 Chirp Filter/C1 FIlter/Sum14 ==
  In1 : Inport
  In2 : Inport  Port=2
  Sum14 : Sum  OutDataTypeStr=single  SampleTime=2.08333333333333e-05  SaturateOnIntegerOverflow=on  InputSameDT=on
  Out1 : Outport
  wires:
  Sum14/1 -> Out1/1
  In2/1 -> Sum14/2
  In1/1 -> Sum14/1

== system AN_Simulink_Model_v1_fil/Auditory Nerve Model/C1 Chirp Filter/C1 FIlter/Sum15 ==
  In1 : Inport
  In2 : Inport  Port=2
  Sum15 : Sum  OutDataTypeStr=single  SampleTime=2.08333333333333e-05  SaturateOnIntegerOverflow=on  InputSameDT=on
  Out1 : Outport
  wires:
  Sum15/1 -> Out1/1
  In2/1 -> Sum15/2
  In1/1 -> Sum15/1

== system AN_Simulink_Model_v1_fil/Auditory Nerve Model/C1 Chirp Filter/C1 FIlter/Sum16 ==
  In1 : Inport
  In2 : Inport  Port=2
  Sum16 : Sum  OutDataTypeStr=single  SampleTime=2.08333333333333e-05  SaturateOnIntegerOverflow=on  InputSameDT=on
  Out1 : Outport
  wires:
  Sum16/1 -> Out1/1
  In2/1 -> Sum16/2
  In1/1 -> Sum16/1

== system AN_Simulink_Model_v1_fil/Auditory Nerve Model/C1 Chirp Filter/C1 FIlter/Sum17 ==
  In1 : Inport
  In2 : Inport  Port=2
  Sum17 : Sum  OutDataTypeStr=single  SampleTime=2.08333333333333e-05  SaturateOnIntegerOverflow=on  InputSameDT=on
  Out1 : Outport
  wires:
  Sum17/1 -> Out1/1
  In2/1 -> Sum17/2
  In1/1 -> Sum17/1

== system AN_Simulink_Model_v1_fil/Auditory Nerve Model/C1 Chirp Filter/C1 FIlter/Sum18 ==
  In1 : Inport
  In2 : Inport  Port=2
  Sum18 : Sum  OutDataTypeStr=single  SampleTime=2.08333333333333e-05  SaturateOnIntegerOverflow=on  InputSameDT=on
  Out1 : Outport
  wires:
  Sum18/1 -> Out1/1
  In2/1 -> Sum18/2
  In1/1 -> Sum18/1

== system AN_Simulink_Model_v1_fil/Auditory Nerve Model/C1 Chirp Filter/C1 FIlter/Sum19 ==
  In1 : Inport
  In2 : Inport  Port=2
  Sum19 : Sum  OutDataTypeStr=single  SampleTime=2.08333333333333e-05  SaturateOnIntegerOverflow=on  InputSameDT=on
  Out1 : Outport
  wires:
  Sum19/1 -> Out1/1
  In2/1 -> Sum19/2
  In1/1 -> Sum19/1

== system AN_Simulink_Model_v1_fil/Auditory Nerve Model/C1 Chirp Filter/C1 FIlter/Sum2 ==
  In1 : Inport
  In2 : Inport  Port=2
  Sum2 : Sum  OutDataTypeStr=single  SampleTime=2.08333333333333e-05  SaturateOnIntegerOverflow=on  InputSameDT=on
  Out1 : Outport
  wires:
  Sum2/1 -> Out1/1
  In2/1 -> Sum2/2
  In1/1 -> Sum2/1

== system AN_Simulink_Model_v1_fil/Auditory Nerve Model/C1 Chirp Filter/C1 FIlter/Sum3 ==
  In1 : Inport
  In2 : Inport  Port=2
  Sum3 : Sum  OutDataTypeStr=single  SampleTime=2.08333333333333e-05  SaturateOnIntegerOverflow=on  InputSameDT=on
  Out1 : Outport
  wires:
  Sum3/1 -> Out1/1
  In2/1 -> Sum3/2
  In1/1 -> Sum3/1

== system AN_Simulink_Model_v1_fil/Auditory Nerve Model/C1 Chirp Filter/C1 FIlter/Sum4 ==
  In1 : Inport
  In2 : Inport  Port=2
  Sum4 : Sum  OutDataTypeStr=single  SampleTime=2.08333333333333e-05  SaturateOnIntegerOverflow=on  InputSameDT=on
  Out1 : Outport
  wires:
  Sum4/1 -> Out1/1
  In2/1 -> Sum4/2
  In1/1 -> Sum4/1

== system AN_Simulink_Model_v1_fil/Auditory Nerve Model/C1 Chirp Filter/C1 FIlter/Sum5 ==
  In1 : Inport
  In2 : Inport  Port=2
  Sum5 : Sum  OutDataTypeStr=single  SampleTime=2.08333333333333e-05  SaturateOnIntegerOverflow=on  InputSameDT=on
  Out1 : Outport
  wires:
  Sum5/1 -> Out1/1
  In2/1 -> Sum5/2
  In1/1 -> Sum5/1

== system AN_Simulink_Model_v1_fil/Auditory Nerve Model/C1 Chirp Filter/C1 FIlter/Sum6 ==
  In1 : Inport
  In2 : Inport  Port=2
  Sum6 : Sum  OutDataTypeStr=single  SampleTime=2.08333333333333e-05  SaturateOnIntegerOverflow=on  InputSameDT=on
  Out1 : Outport
  wires:
  Sum6/1 -> Out1/1
  In2/1 -> Sum6/2
  In1/1 -> Sum6/1

== system AN_Simulink_Model_v1_fil/Auditory Nerve Model/C1 Chirp Filter/C1 FIlter/Sum7 ==
  In1 : Inport
  In2 : Inport  Port=2
  Sum7 : Sum  OutDataTypeStr=single  SampleTime=2.08333333333333e-05  SaturateOnIntegerOverflow=on  InputSameDT=on
  Out1 : Outport
  wires:
  Sum7/1 -> Out1/1
  In2/1 -> Sum7/2
  In1/1 -> Sum7/1

== system AN_Simulink_Model_v1_fil/Auditory Nerve Model/C1 Chirp Filter/C1 FIlter/Sum8 ==
  In1 : Inport
  In2 : Inport  Port=2
  Sum8 : Sum  OutDataTypeStr=single  SampleTime=2.08333333333333e-05  SaturateOnIntegerOverflow=on  InputSameDT=on
  Out1 : Outport
  wires:
  Sum8/1 -> Out1/1
  In2/1 -> Sum8/2
  In1/1 -> Sum8/1

== system AN_Simulink_Model_v1_fil/Auditory Nerve Model/C1 Chirp Filter/C1 FIlter/Sum9 ==
  In1 : Inport
  In2 : Inport  Port=2
  Sum9 : Sum  OutDataTypeStr=single  SampleTime=2.08333333333333e-05  SaturateOnIntegerOverflow=on  InputSameDT=on
  Out1 : Outport
  wires:
  Sum9/1 -> Out1/1
  In2/1 -> Sum9/2
  In1/1 -> Sum9/1

== system AN_Simulink_Model_v1_fil/Auditory Nerve Model/C1 Chirp Filter/Calculate rsigma/Reciprocal1_recip ==
  In1 : Inport
  Reciprocal1_recip : Math  Operator=reciprocal  SampleTime=2.08333333333333e-05  SaturateOnIntegerOverflow=on
  Out1 : Outport
  wires:
  Reciprocal1_recip/1 -> Out1/1
  In1/1 -> Reciprocal1_recip/1

== system AN_Simulink_Model_v1_fil/Auditory Nerve Model/C1 Chirp Filter/Calculate rsigma/Reciprocal_recip ==
  In1 : Inport
  Reciprocal_recip : Math  Operator=reciprocal  SampleTime=2.08333333333333e-05  SaturateOnIntegerOverflow=on
  Out1 : Outport
  wires:
  Reciprocal_recip/1 -> Out1/1
  In1/1 -> Reciprocal_recip/1

== system AN_Simulink_Model_v1_fil/Auditory Nerve Model/C1 Chirp Filter/Calculate rsigma/Subtract ==
  In1 : Inport
  In2 : Inport  Port=2
  Subtract : Sum  Inputs=+-  OutDataTypeStr=single  SampleTime=2.08333333333333e-05  SaturateOnIntegerOverflow=on  InputSameDT=on
  Out1 : Outport
  wires:
  Subtract/1 -> Out1/1
  In2/1 -> Subtract/2
  In1/1 -> Subtract/1

== system AN_Simulink_Model_v1_fil/Auditory Nerve Model/C1 Chirp Filter/Get C1 Coefficients/Add10 ==
  In1 : Inport
  In2 : Inport  Port=2
  Add10 : Sum  OutDataTypeStr=single  SampleTime=2.08333333333333e-05  SaturateOnIntegerOverflow=on  InputSameDT=on
  Out1 : Outport
  wires:
  Add10/1 -> Out1/1
  In2/1 -> Add10/2
  In1/1 -> Add10/1

== system AN_Simulink_Model_v1_fil/Auditory Nerve Model/C1 Chirp Filter/Get C1 Coefficients/Add11 ==
  In1 : Inport
  In2 : Inport  Port=2
  Add11 : Sum  OutDataTypeStr=single  SampleTime=2.08333333333333e-05  SaturateOnIntegerOverflow=on  InputSameDT=on
  Out1 : Outport
  wires:
  Add11/1 -> Out1/1
  In2/1 -> Add11/2
  In1/1 -> Add11/1

== system AN_Simulink_Model_v1_fil/Auditory Nerve Model/C1 Chirp Filter/Get C1 Coefficients/Add12_stage2 ==
  In1 : Inport
  In2 : Inport  Port=2
  Add12_stage2 : Sum  Inputs=+-  OutDataTypeStr=single  SampleTime=2.08333333333333e-05  SaturateOnIntegerOverflow=on  InputSameDT=on
  Out1 : Outport
  wires:
  Add12_stage2/1 -> Out1/1
  In2/1 -> Add12_stage2/2
  In1/1 -> Add12_stage2/1

== system AN_Simulink_Model_v1_fil/Auditory Nerve Model/C1 Chirp Filter/Get C1 Coefficients/Add12_stage3 ==
  In1 : Inport
  In2 : Inport  Port=2
  Add12_stage3 : Sum  Inputs=+-  OutDataTypeStr=single  SampleTime=2.08333333333333e-05  SaturateOnIntegerOverflow=on  InputSameDT=on
  Out1 : Outport
  wires:
  Add12_stage3/1 -> Out1/1
  In2/1 -> Add12_stage3/2
  In1/1 -> Add12_stage3/1

== system AN_Simulink_Model_v1_fil/Auditory Nerve Model/C1 Chirp Filter/Get C1 Coefficients/Add13_stage2 ==
  In1 : Inport
  In2 : Inport  Port=2
  Add13_stage2 : Sum  Inputs=+-  OutDataTypeStr=single  SampleTime=2.08333333333333e-05  SaturateOnIntegerOverflow=on  InputSameDT=on
  Out1 : Outport
  wires:
  Add13_stage2/1 -> Out1/1
  In2/1 -> Add13_stage2/2
  In1/1 -> Add13_stage2/1

== system AN_Simulink_Model_v1_fil/Auditory Nerve Model/C1 Chirp Filter/Get C1 Coefficients/Add13_stage3 ==
  In1 : Inport
  In2 : Inport  Port=2
  Add13_stage3 : Sum  Inputs=+-  OutDataTypeStr=single  SampleTime=2.08333333333333e-05  SaturateOnIntegerOverflow=on  InputSameDT=on
  Out1 : Outport
  wires:
  Add13_stage3/1 -> Out1/1
  In2/1 -> Add13_stage3/2
  In1/1 -> Add13_stage3/1

== system AN_Simulink_Model_v1_fil/Auditory Nerve Model/C1 Chirp Filter/Get C1 Coefficients/Add14_stage2 ==
  In1 : Inport
  In2 : Inport  Port=2
  Add14_stage2 : Sum  Inputs=+-  OutDataTypeStr=single  SampleTime=2.08333333333333e-05  SaturateOnIntegerOverflow=on  InputSameDT=on
  Out1 : Outport
  wires:
  Add14_stage2/1 -> Out1/1
  In2/1 -> Add14_stage2/2
  In1/1 -> Add14_stage2/1

== system AN_Simulink_Model_v1_fil/Auditory Nerve Model/C1 Chirp Filter/Get C1 Coefficients/Add14_stage3 ==
  In1 : Inport
  In2 : Inport  Port=2
  Add14_stage3 : Sum  Inputs=+-  OutDataTypeStr=single  SampleTime=2.08333333333333e-05  SaturateOnIntegerOverflow=on  InputSameDT=on
  Out1 : Outport
  wires:
  Add14_stage3/1 -> Out1/1
  In2/1 -> Add14_stage3/2
  In1/1 -> Add14_stage3/1

== system AN_Simulink_Model_v1_fil/Auditory Nerve Model/C1 Chirp Filter/Get C1 Coefficients/Add15 ==
  In1 : Inport
  In2 : Inport  Port=2
  Add15 : Sum  OutDataTypeStr=single  SampleTime=2.08333333333333e-05  SaturateOnIntegerOverflow=on  InputSameDT=on
  Out1 : Outport
  wires:
  Add15/1 -> Out1/1
  In2/1 -> Add15/2
  In1/1 -> Add15/1

== system AN_Simulink_Model_v1_fil/Auditory Nerve Model/C1 Chirp Filter/Get C1 Coefficients/Add16 ==
  In1 : Inport
  In2 : Inport  Port=2
  Add16 : Sum  OutDataTypeStr=single  SampleTime=2.08333333333333e-05  SaturateOnIntegerOverflow=on  InputSameDT=on
  Out1 : Outport
  wires:
  Add16/1 -> Out1/1
  In2/1 -> Add16/2
  In1/1 -> Add16/1

== system AN_Simulink_Model_v1_fil/Auditory Nerve Model/C1 Chirp Filter/Get C1 Coefficients/Add17 ==
  In1 : Inport
  In2 : Inport  Port=2
  Add17 : Sum  OutDataTypeStr=single  SampleTime=2.08333333333333e-05  SaturateOnIntegerOverflow=on  InputSameDT=on
  Out1 : Outport
  wires:
  Add17/1 -> Out1/1
  In2/1 -> Add17/2
  In1/1 -> Add17/1

== system AN_Simulink_Model_v1_fil/Auditory Nerve Model/C1 Chirp Filter/Get C1 Coefficients/Add4_stage2 ==
  In1 : Inport
  In2 : Inport  Port=2
  Add4_stage2 : Sum  OutDataTypeStr=single  SampleTime=2.08333333333333e-05  SaturateOnIntegerOverflow=on  InputSameDT=on
  Out1 : Outport
  wires:
  Add4_stage2/1 -> Out1/1
  In2/1 -> Add4_stage2/2
  In1/1 -> Add4_stage2/1

== system AN_Simulink_Model_v1_fil/Auditory Nerve Model/C1 Chirp Filter/Get C1 Coefficients/Add4_stage3 ==
  In1 : Inport
  In2 : Inport  Port=2
  Add4_stage3 : Sum  OutDataTypeStr=single  SampleTime=2.08333333333333e-05  SaturateOnIntegerOverflow=on  InputSameDT=on
  Out1 : Outport
  wires:
  Add4_stage3/1 -> Out1/1
  In2/1 -> Add4_stage3/2
  In1/1 -> Add4_stage3/1

== system AN_Simulink_Model_v1_fil/Auditory Nerve Model/C1 Chirp Filter/Get C1 Coefficients/Add5 ==
  In1 : Inport
  In2 : Inport  Port=2
  Add5 : Sum  Inputs=--  OutDataTypeStr=single  SampleTime=2.08333333333333e-05  SaturateOnIntegerOverflow=on  InputSameDT=on
  Out1 : Outport
  wires:
  Add5/1 -> Out1/1
  In2/1 -> Add5/2
  In1/1 -> Add5/1

== system AN_Simulink_Model_v1_fil/Auditory Nerve Model/C1 Chirp Filter/Get C1 Coefficients/Add6 ==
  In1 : Inport
  In2 : Inport  Port=2
  Add6 : Sum  OutDataTypeStr=single  SampleTime=2.08333333333333e-05  SaturateOnIntegerOverflow=on  InputSameDT=on
  Out1 : Outport
  wires:
  Add6/1 -> Out1/1
  In2/1 -> Add6/2
  In1/1 -> Add6/1
